simulink model "milstd_188110Bmodel"  (Simulink 6.0)
settings: Solver=FixedStepDiscrete  SolverMode=SingleTasking  StartTime=0.0  StopTime=4.8*20  RelTol=1e-3
InitFcn:
  | %Initialize variables
  | 
  | milstd = milstd_initmask([gcs '/Simulation Options']);
undefined symbols (not defined in the file or in its folder): figposition, Low, magnitude, slcm
libraries: milstd_library x17, dspsigops x5, commsink2 x4, commchan2 x4, commdigbbndpm2 x2, dspindex x2, commrandsrc2 x1, dspsnks4 x1, simulink x1, dspstat3 x1, dspsrcs4 x1, commeq2 x1
CloseFcn:
  | clear milstd;
settings Model: Creator=arodrigu  LastModifiedBy=arodrigu
settings DataIOCC: LimitDataPoints=off  SaveOutput=off  SaveTime=off  SignalLoggingName=sigsOut
settings OptimizationCC: BooleanDataType=off  InlineInvariantSignals=off
settings DebuggingCC: CheckExecutionContextPreStartOutputMsg=on  CheckExecutionContextRuntimeOutputMsg=on  SolverPrmCheckMsg=none  InheritedTsInSrcMsg=none
settings HardwareCC: TargetHWDeviceType=32-bit Generic  ProdEqTarget=off
settings ModelReferenceCC: UpdateModelReferenceTargets=IfOutOfDate

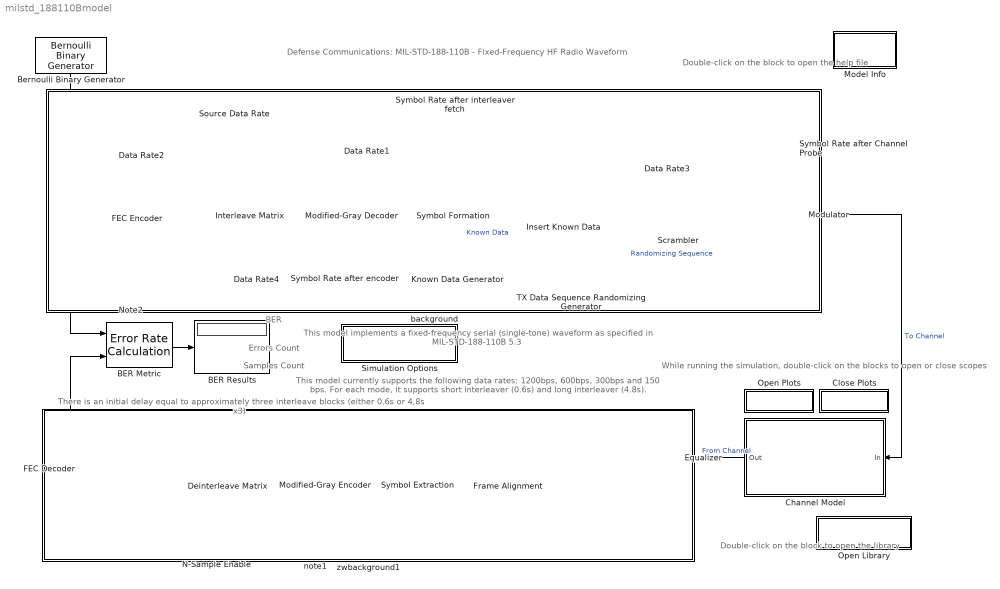
== system milstd_188110Bmodel ==
  note: BER
  note: Errors Count
  note: Samples Count
  note: Defense Communications:
      | MIL-STD-188-110B - Fixed-Frequency HF Radio Waveform
  note: This model currently supports the following data rates: 1200bps,
      | 600bps, 300bps and 150 bps. For each mode, it supports
      | short interleaver (0.6s) and long interleaver (4.8s).
  note: This model implements a fixed-frequency serial (single-tone)
      | waveform as specified in MIL-STD-188-110B 5.3
  note: Double-click on the block
      | to open the help file
  note: While running the simulation,
      | double-click on the blocks
      | to open or close scopes
  note: Double-click on the block
      | to open the library
  note: There is an initial delay equal to approximately
      | three interleave blocks (either 0.6s or 4,8s x3)
  BER Metric : commsink2/Error Rate Calculation  N=34+milstd.rate*milstd.interl*3 % Three interleave blocks plus traceback  st_delay=0  cp_mode=Entire frame  subframe=[]  PMode=Port  WsName=ErrorVec  RsMode2=off  stop=off  numErr=100  maxBits=1e6
  BER Results : Display
  Bernoulli Binary Generator : commrandsrc2/Bernoulli Binary Generator  Orientation=down  P=0.5  seed=61  Ts=1/1200  frameBased=on  sampPerFrame=1200*0.2  orient=off
  Channel Model : Subsystem  Orientation=left  PropExecContextAcrossSSBoundary=on
      mask Display:
      | plot(0,0,100,100,[90,60,70,30,40,10],[50,40,70,40,70,50])
      | text(10,20,'Watterson Fading + AWGN')
  Close Plots : Subsystem  PropExecContextAcrossSSBoundary=on
      settings: OpenFcn=|
      | str1 = 'Equalizer';
      | str2 = 'RX Signal';
      | str3='Equalized Signal';
      | str4 = 'Channel Model';
      | 
      | str5 = 'Main Path Phase Rotation';
      | 
      | str6 = 'Channel Impulse Response';
      | 
      | sdspfscope2([],[],[],'ScopeUpdate',[bdroot '/' str1 '/' str2 ],'CloseFig');
      | sdspfscope2([],[],[],'ScopeUpdate',[bdroot '/' str1 '/' str3 ],'CloseFig');
      | sdspfscope2([],[],[],'ScopeUpdate',[bdroot '/' str4 '/' str5],'CloseFig');
      | sdspfscope2([],[],[],'ScopeUpdate',[bdroot '/' str4 '/' str6],'CloseFig');
      mask Display: disp('Close Scopes');
  Data Rate1 : Subsystem  PropExecContextAcrossSSBoundary=on  mask(Compute Data Rate){N=2}
      mask prompts: N "Bits per symbol:"
      mask Display: disp('Data Rate')
  Data Rate2 : Subsystem  PropExecContextAcrossSSBoundary=on  mask(Compute Data Rate){N=1}
      mask prompts: N "Bits per symbol:"
      mask Display: disp('Data Rate')
  Data Rate3 : Subsystem  PropExecContextAcrossSSBoundary=on  mask(Compute Data Rate){N=3}
      mask prompts: N "Bits per symbol:"
      mask Display: disp('Data Rate')
  Data Rate4 : Subsystem  PropExecContextAcrossSSBoundary=on  mask(Compute Data Rate){N=1}
      mask prompts: N "Bits per symbol:"
      mask Display: disp('Data Rate')
  Deinterleave Matrix : milstd_library/Deinterleave Matrix  Orientation=left
  Equalizer : Subsystem  Orientation=left  PropExecContextAcrossSSBoundary=on
      mask Display: disp('Equalizer:\nLMS Equalizer');
  FEC Decoder : Subsystem  Orientation=left  BlockChoice=Rate 1/2 FEC Decoder  PropExecContextAcrossSSBoundary=on
      settings: AttributesFormatString=%<BlockChoice>  TemplateBlock=milstd_library/FEC Decoder  MemberBlocks=Rate 1/2 FEC Decoder,Rate 1/2 FEC Decoder with Derepetition
  FEC Encoder : Subsystem  BlockChoice=Rate 1/2 FEC Encoder  PropExecContextAcrossSSBoundary=on
      settings: AttributesFormatString=%<BlockChoice>  TemplateBlock=milstd_library/FEC Encoder  MemberBlocks=Rate 1/2 FEC Encoder,Rate 1/2 FEC Encoder with Repetition
  Frame Alignment : milstd_library/Frame Alignment  Orientation=left
  Insert Known Data : milstd_library/Insert Known Data
  Interleave Matrix : milstd_library/Interleave Matrix
  Known Data Generator : milstd_library/Known Data Generator
  Model Info : Subsystem  LoadFcn=slcm LoadBlock;  InitFcn=slcm('UpdateAllCMBlocksInThisModelInit')  PropExecContextAcrossSSBoundary=on  mask(CMBlock){InitialSaveTempField=, InitialBlockCM=None, BlockCM=None, Frame=on, SaveTempField=, DisplayStringWithTags=Info, MaskDisplayString=Info, HorizontalTextAlignment=Center, LeftAlignmentValue=0.5, SourceBlockDiagram=milstd_188110Bmodel, TagMaxNumber=20, CMTag1=, CMTag2=, CMTag3=, CMTag4=, CMTag5=, CMTag6=, CMTag7=, CMTag8=, CMTag9=, CMTag10=, CMTag11=, CMTag12=, CMTag13=, CMTag14=, CMTag15=, CMTag16=, CMTag17=, CMTag18=, CMTag19=, CMTag20=}
      mask help: This block allows revision control information to be displayed within the model.
      settings: CopyFcn=slcm CopyBlock;  DeleteFcn=slcm Cancel;  PostSaveFcn=slcm('UpdateAllCMBlocksInThisModel')  NameChangeFcn=slcm Rename;  OpenFcn=commdemohelp;
      mask Display: text(str2num(LeftAlignmentValue), 0.5, MaskDisplayString, 'HorizontalAlignment', HorizontalTextAlignment)
  Modified-Gray Decoder : milstd_library/Modified-Gray Decoder
  Modified-Gray Encoder : milstd_library/Modified-Gray Encoder  Orientation=left
  Modulator : commdigbbndpm2/M-PSK Modulator Baseband  M=8  InType=Integer  Enc=Binary  Ph=0  numSamp=1
  N-Sample Enable : dspswit3/N-Sample Enable  Orientation=left  N=round(milstd.interl*3/0.2)  ActiveLevel=Low (0)  reset=off  TriggerType=Rising edge  Ts=0.2  DataType=Logical
  Note2 : Subsystem  PropExecContextAcrossSSBoundary=on
      mask Display: disp('Using a configurable\nsubsystem, encoder\n and decoder switch to\nsupport bit repetition\ndepending on data rate')
  Open Library : Subsystem  PropExecContextAcrossSSBoundary=on
      settings: OpenFcn=open('milstd_library.mdl');
      mask Display: disp('MIL-STD-188-110B\nLibrary')
  Open Plots : Subsystem  PropExecContextAcrossSSBoundary=on
      settings: OpenFcn=|
      | str1 = 'Equalizer';
      | str2 = 'RX Signal';
      | str3='Equalized Signal';
      | str4 = 'Channel Model';
      | 
      | str5 = 'Main Path Phase Rotation';
      | 
      | str6 = 'Channel Impulse Response';
      | 
      | sdspfscope2([],[],[],'ScopeUpdate',[bdroot '/' str1 '/' str2 ],'OpenFig');
      | sdspfscope2([],[],[],'ScopeUpdate',[bdroot '/' str1 '/' str3 ],'OpenFig');
      | sdspfscope2([],[],[],'ScopeUpdate',[bdroot '/'  str4 '/' str5 ],'OpenFig');
      | sdspfscope2([],[],[],'ScopeUpdate',[bdroot '/'  str4 '/' str6 ],'OpenFig');
      mask Display: disp('Open Scopes');
  Scrambler : milstd_library/Scrambler
  Simulation Options : Subsystem  PropExecContextAcrossSSBoundary=on  mask(Simulation options){infRate=1200, intLength=0.6}
      mask prompts: infRate "Information Rate (bps):"; intLength "Interleaver length (s):"
      mask help:
      | Select the different options for the simulation.
      |
      | This model currently supports the following data rates: 1200 bps, 600 bps, 300 bps and 150 bps.
      |
      | For each data rate, the model implements short (0.6s) and long (4.8s) interleaver.
      mask init:
      | milstd = milstd_initmask(gcb);
      | assignin('base','milstd',milstd);
      settings: AttributesFormatString=Data Rate = %<infRate> bps\nInterleaver Length = %<intLength> s
      mask Help: eval('commdemohelp;');
      mask StyleString: popup(1200|600|300|150),popup(4.8|0.6)
      mask Display: disp('Simulation\nOptions')
  Source Data Rate : Display
  Symbol Extraction : milstd_library/Symbol Extraction  Orientation=left
  Symbol Formation : milstd_library/Symbol Formation
  Symbol Rate after Channel Probe : Display
  Symbol Rate after encoder : Display
  Symbol Rate after interleaver fetch : Display
  TX Data Sequence Randomizing Generator : milstd_library/Data Sequence Randomizing Generator
  background : Subsystem  PropExecContextAcrossSSBoundary=on
      mask Display: disp('')
  note1 : Subsystem  PropExecContextAcrossSSBoundary=on
      mask Display: disp('Need to reset encoder after\n initial frame delay introduced\n by the deinterleaver')
  zwbackground1 : Subsystem  PropExecContextAcrossSSBoundary=on
      mask Display: disp('')
  wires:
  FEC Encoder/1(outCodedBits) -> Interleave Matrix/1, Data Rate4/1(In1)
  Interleave Matrix/1 -> Data Rate1/1(In1), Modified-Gray Decoder/1
  Modified-Gray Decoder/1 -> Symbol Formation/1
  Symbol Formation/1 -> Insert Known Data/1
  Known Data Generator/1 -> Insert Known Data/2  "Known Data"
  Data Rate2/1(Out1) -> Source Data Rate/1
  Symbol Extraction/1 -> Modified-Gray Encoder/1
  FEC Decoder/1(outBits) -> BER Metric/2
  BER Metric/1 -> BER Results/1
  Bernoulli Binary Generator/1 -> Data Rate2/1(In1), BER Metric/1, FEC Encoder/1(inBits)
  N-Sample Enable/1 -> FEC Decoder/2(Rst)
  Insert Known Data/1 -> Data Rate3/1(In1), Scrambler/1
  Data Rate1/1(Out1) -> Symbol Rate after interleaver fetch/1
  Data Rate3/1(Out1) -> Symbol Rate after Channel Probe/1
  Data Rate4/1(Out1) -> Symbol Rate after encoder/1
  Scrambler/1 -> Modulator/1
  TX Data Sequence Randomizing Generator/1 -> Scrambler/2  "Randomizing Sequence"
  Deinterleave Matrix/1 -> FEC Decoder/1(inCodedBits)
  Modified-Gray Encoder/1 -> Deinterleave Matrix/1
  Equalizer/1(Data_hard) -> Frame Alignment/1
  Frame Alignment/1 -> Symbol Extraction/1
  Modulator/1 -> Channel Model/1(In)  "To Channel"
  Channel Model/1(Out) -> Equalizer/1(RxData)  "From Channel"

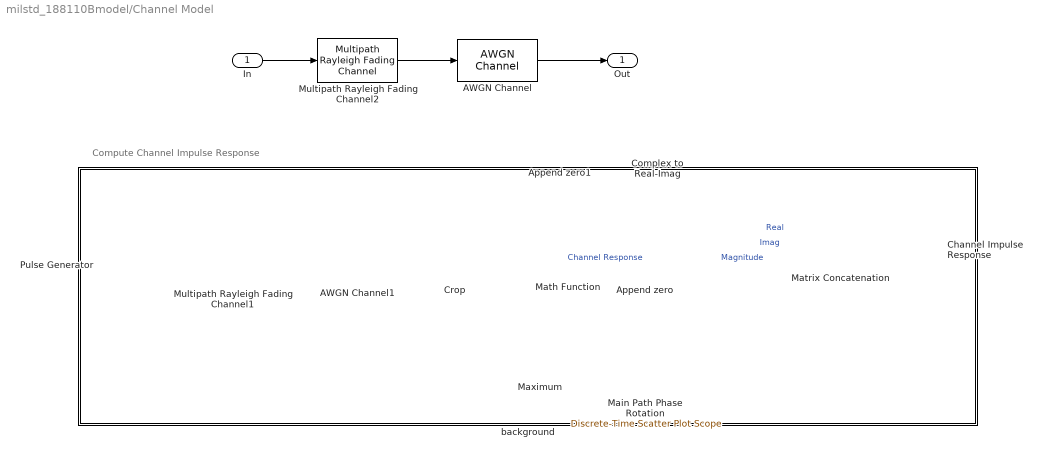
== system milstd_188110Bmodel/Channel Model ==
  note: Compute Channel Impulse Response
  In : Inport  LatchInput=off
  AWGN Channel : commchan2/AWGN Channel  seed=67  noiseMode="Signal to noise ratio  (Es/No)"  EbNodB=10  EsNodB=27  SNRdB=10  bitsPerSym=1  Ps=1  Tsym=1/2400  variance=1
  AWGN Channel1 : commchan2/AWGN Channel  seed=67  noiseMode="Signal to noise ratio  (Es/No)"  EbNodB=10  EsNodB=27  SNRdB=10  bitsPerSym=1  Ps=1  Tsym=1/2400  variance=1
  Append zero : dspsigops/Zero Pad  padSigAt=Beginning  zpadAlong=Columns  padNumOutRowsSpecMethod=User-specified  numOutRows=9  padNumOutColsSpecMethod=User-specified  numOutCols=1  trunc_flag=None
  Append zero1 : dspsigops/Zero Pad  padSigAt=Beginning  zpadAlong=Columns  padNumOutRowsSpecMethod=User-specified  numOutRows=9  padNumOutColsSpecMethod=User-specified  numOutCols=1  trunc_flag=None
  Channel Impulse Response : dspsnks4/Vector Scope  ScopeProperties=off  Domain=User-defined  HorizSpan=1  DisplayProperties=off  AxisGrid=on  Memory=off  FrameNumber=off  AxisLegend=on  AxisZoom=off  OpenScopeAtSimStart=on  OpenScopeImmediately=off  FigPos="figposition([6    61    57    28])"  AxisProperties=on  XUnits=Hertz  XRange=[0...Fs/2]  InheritXIncr=off  XIncr=1  XLabel=Channel Impulse Response  YUnits=dB  YLabel=Amplitude  LineProperties=off  LineMarkers=*|*|o  LineColors=[0 0 1]|[1 0 0]|[0 0 0]
      settings: YMin=-2  YMax=2
  Complex to Real-Imag : ComplexToRealImag
  Crop : dspsigops/Zero Pad  padSigAt=End  zpadAlong=Columns  padNumOutRowsSpecMethod=User-specified  numOutRows=8  padNumOutColsSpecMethod=User-specified  numOutCols=1  trunc_flag=None
  Main Path Phase Rotation : commsink2/Discrete-Time Scatter Plot Scope  Tag=ScatterPlot  sampPerSymb=1  offsetEye=0  numTraces=100  numNewFrames=5  LineMarkers=.  LineColors=b  fading=on  render=on  AxisGrid=on  xMin=-2  xMax=2  yMin=-2  yMax=2  inphaseLabel=Main Path Phase Rotation  quadratureLabel=.  openScopeAtSimStart=on  FrameNumber=off  FigPos="figposition([65    61    24    32])"  figTitle=.  numLinesMax=8  block_type_=scatter
  Math Function : Math  Operator=magnitude^2  SaturateOnIntegerOverflow=on
  Matrix Concatenation : simulink/Math Operations/Matrix Concatenation  numInports=3  catMethod=Horizontal
  Maximum : dspstat3/Maximum  fcn=Value  reset=None  roundingMode=Floor  overflowMode=off
  Multipath Rayleigh Fading Channel1 : commchan2/Multipath Rayleigh Fading Channel  Fd=0.075  simTs=1/2400  delayVec=[0 2e-3]  gainVecdB=[0 0]  normGain=off  Seed=73
  Multipath Rayleigh Fading Channel2 : commchan2/Multipath Rayleigh Fading Channel  Fd=0.075  simTs=1/2400  delayVec=[0 2e-3]  gainVecdB=[0 0]  normGain=off  Seed=73
  Pulse Generator : Subsystem  PropExecContextAcrossSSBoundary=on
      mask Display: plot(0,0,45,100,[5 10 10 10 40],[0 0 60 0 0]+20)
  background : Subsystem  PropExecContextAcrossSSBoundary=on
      mask Display: disp('')
  Out : Outport
  wires:
  In/1 -> Multipath Rayleigh Fading Channel2/1
  Crop/1 -> Maximum/1, Math Function/1, Append zero1/1
  Math Function/1 -> Append zero/1  "Channel Response"
  Multipath Rayleigh Fading Channel2/1 -> AWGN Channel/1
  Multipath Rayleigh Fading Channel1/1 -> AWGN Channel1/1
  AWGN Channel/1 -> Out/1
  AWGN Channel1/1 -> Crop/1
  Append zero/1 -> Matrix Concatenation/3  "Magnitude"
  Maximum/1 -> Main Path Phase Rotation/1
  Pulse Generator/1(Out1) -> Multipath Rayleigh Fading Channel1/1
  Append zero1/1 -> Complex to Real-Imag/1
  Complex to Real-Imag/1 -> Matrix Concatenation/1  "Real"
  Complex to Real-Imag/2 -> Matrix Concatenation/2  "Imag"
  Matrix Concatenation/1 -> Channel Impulse Response/1

== system milstd_188110Bmodel/Close Plots ==
  note: This subsystem is empty

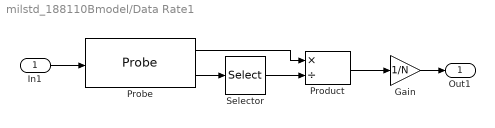
== system milstd_188110Bmodel/Data Rate1 ==
  In1 : Inport  LatchInput=off
  Gain : Gain  Gain=1/N  SaturateOnIntegerOverflow=on
  Probe : Probe  ProbeComplexSignal=off
  Product : Product  Inputs=*/  SaturateOnIntegerOverflow=on
  Selector : Selector  InputPortWidth=2
  Out1 : Outport
  wires:
  Gain/1 -> Out1/1
  Probe/1 -> Product/1
  Probe/2 -> Selector/1
  Selector/1 -> Product/2
  In1/1 -> Probe/1
  Product/1 -> Gain/1

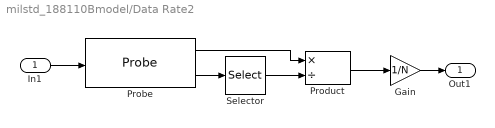
== system milstd_188110Bmodel/Data Rate2 ==
  In1 : Inport  LatchInput=off
  Gain : Gain  Gain=1/N  SaturateOnIntegerOverflow=on
  Probe : Probe  ProbeComplexSignal=off
  Product : Product  Inputs=*/  SaturateOnIntegerOverflow=on
  Selector : Selector  InputPortWidth=2
  Out1 : Outport
  wires:
  Product/1 -> Gain/1
  In1/1 -> Probe/1
  Selector/1 -> Product/2
  Probe/2 -> Selector/1
  Probe/1 -> Product/1
  Gain/1 -> Out1/1

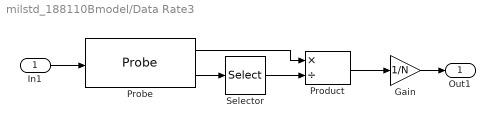
== system milstd_188110Bmodel/Data Rate3 ==
  In1 : Inport  LatchInput=off
  Gain : Gain  Gain=1/N  SaturateOnIntegerOverflow=on
  Probe : Probe  ProbeComplexSignal=off
  Product : Product  Inputs=*/  SaturateOnIntegerOverflow=on
  Selector : Selector  InputPortWidth=2
  Out1 : Outport
  wires:
  Product/1 -> Gain/1
  In1/1 -> Probe/1
  Selector/1 -> Product/2
  Probe/2 -> Selector/1
  Probe/1 -> Product/1
  Gain/1 -> Out1/1

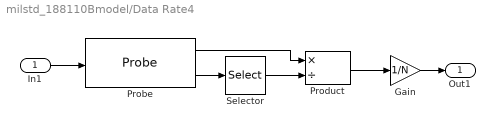
== system milstd_188110Bmodel/Data Rate4 ==
  In1 : Inport  LatchInput=off
  Gain : Gain  Gain=1/N  SaturateOnIntegerOverflow=on
  Probe : Probe  ProbeComplexSignal=off
  Product : Product  Inputs=*/  SaturateOnIntegerOverflow=on
  Selector : Selector  InputPortWidth=2
  Out1 : Outport
  wires:
  Product/1 -> Gain/1
  In1/1 -> Probe/1
  Selector/1 -> Product/2
  Probe/2 -> Selector/1
  Probe/1 -> Product/1
  Gain/1 -> Out1/1

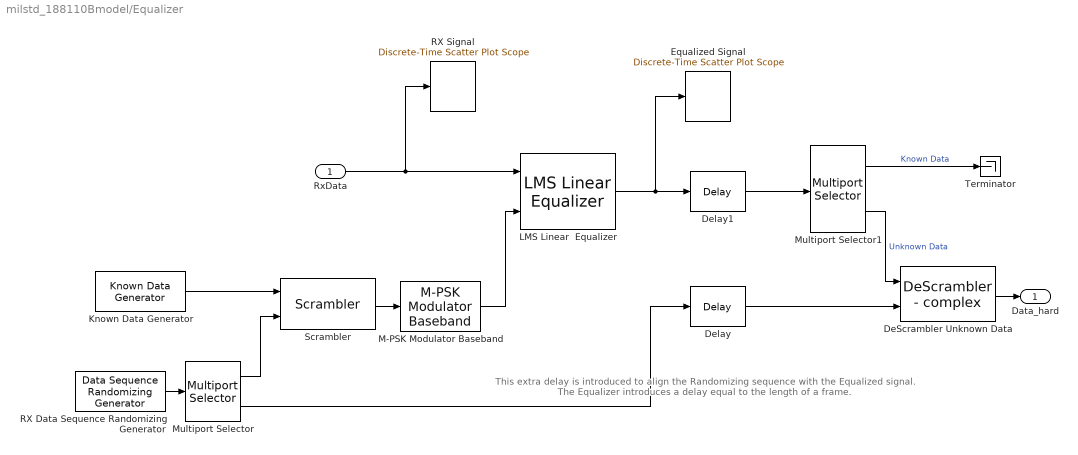
== system milstd_188110Bmodel/Equalizer ==
  note: This extra delay is introduced to align the
      | Randomizing sequence with the Equalized signal.
      | The Equalizer introduces a delay equal to the length
      | of a frame.
  RxData : Inport  LatchInput=off
  DeScrambler Unknown Data : milstd_library/DeScrambler - complex
  Delay : dspsigops/Delay  dly_unit=Samples  delay=20  ic_detail=off  dif_ic_for_ch=off  dif_ic_for_dly=off  ic=0  reset_popup=None
  Delay1 : dspsigops/Delay  dly_unit=Samples  delay=40-1  ic_detail=off  dif_ic_for_ch=off  dif_ic_for_dly=off  ic=0  reset_popup=None
  Equalized Signal : commsink2/Discrete-Time Scatter Plot Scope  Tag=ScatterPlot  sampPerSymb=1  offsetEye=0  numTraces=160  numNewFrames=40  LineMarkers=.  LineColors=b  fading=on  render=on  AxisGrid=on  xMin=-1.29510330913857  xMax=1.33819643567585  yMin=-1.33057365332797  yMax=1.30272609148645  inphaseLabel=After Equalizer (To Decoding)  quadratureLabel=.  openScopeAtSimStart=on  FrameNumber=off  FigPos="figposition([40    11    32    43])"  figTitle=.  numLinesMax=8  block_type_=scatter
  Known Data Generator : milstd_library/Known Data Generator
  LMS Linear  Equalizer : commeq2/LMS Linear  Equalizer  nTaps=16  nSamp=1  sigConst=pskmod([0:7],8) % 8-PSK modulation  delay=1  stepSize=0.01  leakage=1  initWeights=[1 zeros(1,15)]  mode=off  outErr=off  outWeights=off
  M-PSK Modulator Baseband : commdigbbndpm2/M-PSK Modulator Baseband  M=8  InType=Integer  Enc=Binary  Ph=0  numSamp=1
  Multiport Selector : dspindex/Multiport Selector  rowsOrCols=Rows  idxCellArray={[1:20],[21:40] }  idxErrMode=Clip Index
  Multiport Selector1 : dspindex/Multiport Selector  rowsOrCols=Rows  idxCellArray={ [1:20],[21:40]}  idxErrMode=Clip Index
  RX Data Sequence Randomizing Generator : milstd_library/Data Sequence Randomizing Generator
  RX Signal : commsink2/Discrete-Time Scatter Plot Scope  Tag=ScatterPlot  sampPerSymb=1  offsetEye=0  numTraces=160  numNewFrames=40  LineMarkers=.  LineColors=b  fading=on  render=on  AxisGrid=on  xMin=-1.91692231790696  xMax=1.9414795542373  yMin=-1.93559587800639  yMax=1.92280599413788  inphaseLabel=Before Equalizer (From Channel)  quadratureLabel=.  openScopeAtSimStart=on  FrameNumber=off  FigPos="figposition([6    11    32    43])"  figTitle=.  numLinesMax=8  block_type_=scatter
  Scrambler : milstd_library/Scrambler
  Terminator : Terminator
  Data_hard : Outport
  wires:
  DeScrambler Unknown Data/1 -> Data_hard/1
  RX Data Sequence Randomizing Generator/1 -> Multiport Selector/1
  Known Data Generator/1 -> Scrambler/1
  Multiport Selector/1 -> Scrambler/2
  Multiport Selector/2 -> Delay/1
  Scrambler/1 -> M-PSK Modulator Baseband/1
  Delay/1 -> DeScrambler Unknown Data/2
  RxData/1 -> LMS Linear  Equalizer/1, RX Signal/1
  LMS Linear  Equalizer/1 -> Delay1/1, Equalized Signal/1
  Multiport Selector1/2 -> DeScrambler Unknown Data/1  "Unknown Data"
  Multiport Selector1/1 -> Terminator/1  "Known Data"
  M-PSK Modulator Baseband/1 -> LMS Linear  Equalizer/2
  Delay1/1 -> Multiport Selector1/1

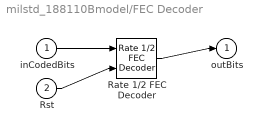
== system milstd_188110Bmodel/FEC Decoder ==
  inCodedBits : Inport  LatchInput=off
  Rst : Inport  Port=2  LatchInput=off
  Rate 1/2 FEC Decoder : milstd_library/Rate 1//2 FEC Decoder
  outBits : Outport
  wires:
  inCodedBits/1 -> Rate 1/2 FEC Decoder/1
  Rst/1 -> Rate 1/2 FEC Decoder/2
  Rate 1/2 FEC Decoder/1 -> outBits/1

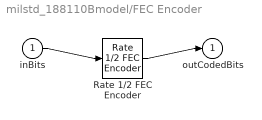
== system milstd_188110Bmodel/FEC Encoder ==
  inBits : Inport  LatchInput=off
  Rate 1/2 FEC Encoder : milstd_library/Rate 1//2 FEC Encoder
  outCodedBits : Outport
  wires:
  inBits/1 -> Rate 1/2 FEC Encoder/1
  Rate 1/2 FEC Encoder/1 -> outCodedBits/1

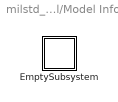
== system milstd_188110Bmodel/Model Info ==
  EmptySubsystem : Subsystem  PropExecContextAcrossSSBoundary=on

== system milstd_188110Bmodel/Note2 ==

== system milstd_188110Bmodel/Open Library ==
  note: This subsystem is intentionally left empty

== system milstd_188110Bmodel/Open Plots ==
  note: This subsystem is empty

== system milstd_188110Bmodel/Simulation Options ==
  note: This subsystem is empty

== system milstd_188110Bmodel/background ==
  note: This subsystem is empty

== system milstd_188110Bmodel/note1 ==

== system milstd_188110Bmodel/zwbackground1 ==
  note: This subsystem is empty

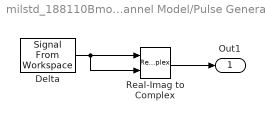
== system milstd_188110Bmodel/Channel Model/Pulse Generator ==
  Delta : dspsrcs4/Signal From Workspace  X=[1; zeros(39,1)]  Ts=1/2400  nsamps=40  OutputAfterFinalValue=Cyclic repetition
  Real-Imag to Complex : RealImagToComplex
  Out1 : Outport
  wires:
  Delta/1 -> Real-Imag to Complex/1, Real-Imag to Complex/2
  Real-Imag to Complex/1 -> Out1/1

== system milstd_188110Bmodel/Channel Model/background ==
  note: This subsystem is empty

== system milstd_188110Bmodel/Model Info/EmptySubsystem ==
